simulink model "Copy_of_eCS_Algo_Simulation_2015b"  (R2015b)
settings: Solver=ode1  StartTime=0.0  StopTime=3  FixedStep=1/80000  RelTol=1e-3
PreLoadFcn:
  | if exist('tl_preloadfcn','file'), tl_preloadfcn(gcs,402); end
PostLoadFcn:
  | , if any(exist('dsrtsu_mdlpostloadfcn', 'file') == [2, 3, 6]), try dsrtsu_mdlpostloadfcn('Execute', bdroot); catch fprintf('Error in PostLoadFcn (dsrtsu_mdlpostloadfcn) for model "%s":\n %s\n', bdroot, lasterr); end, end,
  | if exist('tl_postloadfcn','file'), tl_postloadfcn(gcs,402); end
InitFcn:
  | if exist('tlds_init','file'), tlds_init(gcs); end
StartFcn:
  | if exist('tlds_start','file'), tlds_start(gcs); end
StopFcn:
  | if exist('tlds_stop','file'), tlds_stop(gcs); end
model workspace (MAT data in the model file):
  au8PrevExecProfile = [0 0 0 0 0 0]
values from neighbouring files (symbols this model uses):
  AccSensor = 5    [Parameter_eCS_Algo.m]
  AlgoType = 0    [Parameter_eCS_Algo.m]
  Cxy = 1*0.017    (= 0.017)    [Acc_Init_SelV1.m]
  Cxz = 1*0.017    (= 0.017)    [Acc_Init_SelV1.m]
  Cyx = 1*0.017    (= 0.017)    [Acc_Init_SelV1.m]
  Cyz = 1*0.017    (= 0.017)    [Acc_Init_SelV1.m]
  Czx = 1*0.017    (= 0.017)    [Acc_Init_SelV1.m]
  Czy = 1*0.017    (= 0.017)    [Acc_Init_SelV1.m]
  Forced_Oscillation = 0    [Parameter_eCS_Algo.m]    (also in run_Rotation_sim.m = run)
  FreqTemperature = 10    [Acc_Init_SelV1.m]
  MaxSensorOffset = 0.3    [Acc_Init_SelV1.m]
  Mean_x_noise = 4e-3    (= 0.004)    [Acc_Init_SelV1.m]
  Mean_y_noise = 4e-3    (= 0.004)    [Acc_Init_SelV1.m]
  Mean_z_noise = 4e-3    (= 0.004)    [Acc_Init_SelV1.m]
  ODR = 8000    [Acc_Init_SelV1.m]
  offsetcorrection_on_off = 0    [Parameter_eCS_Algo.m]
  phi_pulse_rotation = 0    [Parameter_eCS_Algo.m]    (also in run_Rotation_sim.m = angle)
  pulsetype = 2    [Parameter_eCS_Algo.m]    (also in run_simulation.m = j; run_simulation_ActiveX.m = j)
  Range = 4    [Acc_Init_SelV1.m]
  TempBias = 0    [Acc_Init_SelV1.m]
  TemperatureAmp = 0    [Acc_Init_SelV1.m]
  Var_x_noise = 1.84e-9    (= 1.84e-09)    [Acc_Init_SelV1.m]
  Var_y_noise = 2.025e-09    [Acc_Init_SelV1.m]
  Var_z_noise = 1.374e-09    [Acc_Init_SelV1.m]
  w_x = 2*pi*F_x    (= 376.991118431)    [Acc_Init_SelV1.m]
  w_y = 2*pi*F_y    (= 376.991118431)    [Acc_Init_SelV1.m]
  w_z = 2*pi*F_z    (= 376.991118431)    [Acc_Init_SelV1.m]
  x_max_temp_drift = 0.061    [Acc_Init_SelV1.m]
  x_offset_enable = 0    [Acc_Init_SelV1.m]
  x_run_to_run_drift = 0.0    (= 0)    [Acc_Init_SelV1.m]
  x_temp_co_drift = 0.000    (= 0)    [Acc_Init_SelV1.m]
  Xi_x = 0.7    [Acc_Init_SelV1.m]
  Xi_y = 0.7    [Acc_Init_SelV1.m]
  Xi_z = 0.7    [Acc_Init_SelV1.m]
  y_max_temp_drift = 0.061    [Acc_Init_SelV1.m]
  y_offset_enable = 0    [Acc_Init_SelV1.m]
  y_run_to_run_drift = 0.0    (= 0)    [Acc_Init_SelV1.m]
  y_temp_co_drift = 0.000    (= 0)    [Acc_Init_SelV1.m]
  z_max_temp_drift = 0.13    [Acc_Init_SelV1.m]
  z_offset_enable = 0    [Acc_Init_SelV1.m]
  z_run_to_run_drift = 0.0    (= 0)    [Acc_Init_SelV1.m]
  z_temp_co_drift = 0.000    (= 0)    [Acc_Init_SelV1.m]
undefined symbols (not defined in the file or in its folder): controller_sample_rate, ddv, DiscIntNeverNeededParam, ECE_L_0_x, ECE_L_0_y, ECE_L_0_z, ECE_L_45_time, ECE_L_45_x, ECE_L_45_y, ECE_L_45_z, FMVSS_45_time, FMVSS_45_x, FMVSS_45_y, FMVSS_45_z, gmw_roada_x__m_s__, gmw_roada_y__m_s__, gmw_roadtime_2kHz, KSF_50_a_x, KSF_50_a_y, KSF_50_time, KSG_30_a_x, KSG_30_a_y, KSG_30_time, Meldorf_HindenburgstraAcceleration_x__m_s_2_, Meldorf_HindenburgstraAcceleration_y__m_s_2_, Meldorf_HindenburgstraAcceleration_z__m_s_2_, Meldorf_HindenburgstraTime__s_, pulse_FF27, pulse_MPDB, pulse_ODB40, pulse_ODB64, pulse_USNCAP, pulsetime_FF27, pulsetime_MPDB, pulsetime_ODB40, pulsetime_ODB64, pulsetime_USNCAP, Rauasphalt_60_a_x, Rauasphalt_60_a_y, Rauasphalt_60_time, sigbuilder_block, TimeArray, VW_416_2kHza_x_2kHz, VW_416_2kHza_y_2kHz, VW_416_2kHztime_2kHz
libraries: simulink x40, tllib x10, tl_autosar_lib x7, simulink_extras x5, LIB_TF_G_111 x2, LIB_TF_G_12_StepControl x2, LIB_TF_G_112 x1, dspsigops x1
(part 2 of 9)

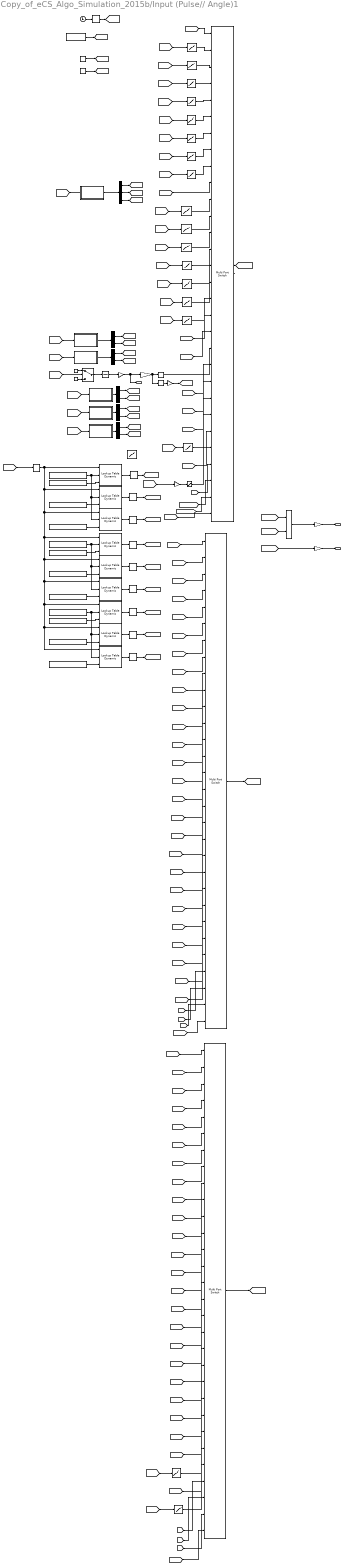
== system Copy_of_eCS_Algo_Simulation_2015b/Input (Pulse// Angle)1 ==
  note: pulse tables must begin and end with 0 !!!!!!!
  -1.0 : Constant  Value=-1
  BMW QV72003-3 no-fire lower : Lookup_n-D  NumberOfTableDimensions=1  BreakpointsForDimension1=[-0.011 0.00 0.020 0.045 0.059]  Table=[0 0 11.0 11.0 0]  ExtrapMethod=Clip  UseLastTableValue=on  InternalRulePriority=Speed  RndMeth=Simplest  InputSameDT=on
  BMW QV72003-3 no-fire upper : Lookup_n-D  NumberOfTableDimensions=1  BreakpointsForDimension1=[0 0.027 0.059 0.085]  Table=[0 16.2 16.2 0]  ExtrapMethod=Clip  UseLastTableValue=on  InternalRulePriority=Speed  RndMeth=Simplest  InputSameDT=on
  Clock : Clock
  Constant : Constant  Value=TimeArray
  Constant1 : Constant  Value=ECE_L_0_x
  Constant10 : Constant  Value=FMVSS_45_z
  Constant11 : Constant  Value=FMVSS_45_y
  Constant2 : Constant  Value=ECE_L_0_z
  Constant3 : Constant  Value=ECE_L_0_y
  Constant4 : Constant  Value=ECE_L_45_time
  Constant5 : Constant  Value=ECE_L_45_x
  Constant6 : Constant  Value=ECE_L_45_z
  Constant7 : Constant  Value=ECE_L_45_y
  Constant8 : Constant  Value=FMVSS_45_time
  Constant9 : Constant  Value=FMVSS_45_x
  Demux1 : Demux  Outputs=3
  Demux{2..6} (5 alike) : Demux  Outputs=2
  Discrete-Time Integrator4 : DiscreteIntegrator  gainval=1  InitialConditionSetting=State (most efficient)  SampleTime=-1  UpperSaturationLimit=0.3 * 9.81  LowerSaturationLimit=-0.3 * 9.81  ICPrevOutput=DiscIntNeverNeededParam  ICPrevScaledInput=DiscIntNeverNeededParam
  Gain : Gain  Gain=-1
  Lookup Table Dynamic{,1..8} (9 alike) : simulink/Lookup Tables/Lookup Table Dynamic  LookUpMeth=Interpolation-Use End Values  OutDataTypeStr=fixdt('double')  OutputDataTypeScalingMode=Specify via dialog  OutDataType=fixdt('double')  OutScaling=[]  DoSatur=off
  Multiport Switch1 : MultiPortSwitch  Inputs=28  DataPortForDefault=Additional data port
  Multiport Switch2 : MultiPortSwitch  Inputs=28  DataPortForDefault=Additional data port
  Multiport Switch3 : MultiPortSwitch  Inputs=28  DataPortForDefault=Additional data port
  Mux1 : Mux  Inputs=2
  Puls_BMW_KSF_50 : Subsystem
  Puls_BMW_KSG_30 : Subsystem
  "Puls_BMW_Rauasphalt_60 " : Subsystem
  Puls_GWM_road_C.Morgan : Subsystem
  Puls_Kopfsteinpflaster Meldorf Hindenburgstrasse : Subsystem
  Puls_VW416_Atlas_C.Morgan : Subsystem
  Pulse table FF27 (g) : Lookup  InputValues=pulsetime_FF27  Table=pulse_FF27  LookUpMeth=Interpolation-Use End Values
  Pulse table MPDB (g) : Lookup  InputValues=pulsetime_MPDB  Table=pulse_MPDB  LookUpMeth=Interpolation-Use End Values
  Pulse table ODB40 (g) : Lookup  InputValues=pulsetime_ODB40  Table=pulse_ODB40  LookUpMeth=Interpolation-Use End Values
  Pulse table ODB64 (g) : Lookup  InputValues=pulsetime_ODB64  Table=pulse_ODB64  LookUpMeth=Interpolation-Use End Values
  Pulse table USNCAP (g) : Lookup  InputValues=pulsetime_USNCAP  Table=pulse_USNCAP  LookUpMeth=Interpolation-Use End Values
  Rate Transition{,1,3..10} (10 alike) : RateTransition
  Rate Transition2 : RateTransition  OutPortSampleTime=1/2000
  Saturation : Saturate  UpperLimit=5  LowerLimit=0
  Sin1 : Trigonometry  Operator=cos
  Sin2 : Trigonometry
  Switch : Switch  Criteria=u2 > Threshold  Threshold=36
  crash angle in rad : Gain  Gain=2*pi/360
  g in m/s² : Gain  Gain=9.807
  g in m/s²1 : Gain  Gain=9.807
  "g-lock \" must lock\" - 6g/s - 0.45g" : Lookup_n-D  NumberOfTableDimensions=1  BreakpointsForDimension1=[0 0.075 0.3 0.4]  Table=[0 0.45 0.45 0]  ExtrapMethod=Clip  UseLastTableValue=on  InternalRulePriority=Speed  RndMeth=Simplest  InputSameDT=on
  "g-lock \" no lock\" - 6g/s - 0.3g" : Lookup_n-D  NumberOfTableDimensions=1  BreakpointsForDimension1=[0 0.050 0.5 0.6]  Table=[0 0.3 0.3 0]  ExtrapMethod=Clip  UseLastTableValue=on  InternalRulePriority=Speed  RndMeth=Simplest  InputSameDT=on
  g-lock Crash - 2000g/s - 30g : Lookup_n-D  NumberOfTableDimensions=1  BreakpointsForDimension1=[0 0.015 0.055 0.08]  Table=[0 30 30 0]  ExtrapMethod=Clip  UseLastTableValue=on  InternalRulePriority=Speed  RndMeth=Simplest  InputSameDT=on
  g-lock ECE - 150g/s - 0.45g : Lookup_n-D  NumberOfTableDimensions=1  BreakpointsForDimension1=[0 0.003 0.3 0.4]  Table=[0 0.45 0.45 0]  ExtrapMethod=Clip  UseLastTableValue=on  InternalRulePriority=Speed  RndMeth=Simplest  InputSameDT=on
  g-lock ECE - 25g/s - 0.45g : Lookup_n-D  NumberOfTableDimensions=1  BreakpointsForDimension1=[0 0.018 0.3 0.4]  Table=[0 0.45 0.45 0]  ExtrapMethod=Clip  UseLastTableValue=on  InternalRulePriority=Speed  RndMeth=Simplest  InputSameDT=on
  g-lock ECE - 25g/s - 0.45g custom : Lookup_n-D  NumberOfTableDimensions=1  BreakpointsForDimension1=[0 0.1 0.10001 1]  Table=[0 0 1 1]  ExtrapMethod=Clip  UseLastTableValue=on  InternalRulePriority=Speed  RndMeth=Simplest  InputSameDT=on
  g-lock ECE - 25g/s - 0.45g custom1 : Lookup_n-D  NumberOfTableDimensions=1  BreakpointsForDimension1=[0,0.018,0.3,0.4,0.6,0.618,1,1.1,3,3.018,3.05,3.1,3.118,3.5,3.6,4,4.018,4.2,4.3,8,8.018,8.1,8.15,9,9.018,9.3,9.4,10]  Table=[0,0.45,0.45,0,0,0.45,0.45,0,0,0.45,0.45,0,0.45,0.45,0,0,0.45,0.45,0,0,0.45,0.45,0,0,0.45,0.45,0,0]  ExtrapMethod=Clip  UseLastTableValue=on  InternalRulePriority=Speed  RndMeth=Simplest  InputSameDT=on
  g-lock FMVSS  - 16g/s - 0,7g : Lookup_n-D  NumberOfTableDimensions=1  BreakpointsForDimension1=[0 0.04375 0.3 0.4]  Table=[0 0.7 0.7 0]  ExtrapMethod=Clip  UseLastTableValue=on  InternalRulePriority=Speed  RndMeth=Simplest  InputSameDT=on
  g-lock FMVSS - 70g/s - 0.7g : Lookup_n-D  NumberOfTableDimensions=1  BreakpointsForDimension1=[0 0.01 0.3 0.4]  Table=[0 0.7 0.7 0]  ExtrapMethod=Clip  UseLastTableValue=on  InternalRulePriority=Speed  RndMeth=Simplest  InputSameDT=on
  g-lock Vollbremsung - 4g/s - 1g : Lookup_n-D  NumberOfTableDimensions=1  BreakpointsForDimension1=[0 0.25 0.9745 1.2]  Table=[0 1 1 0]  ExtrapMethod=Clip  UseLastTableValue=on  InternalRulePriority=Speed  RndMeth=Simplest  InputSameDT=on
  g_rate : Gain  Gain=5
  generic rollover : Lookup_n-D  NumberOfTableDimensions=1  BreakpointsForDimension1=[0 15 16 20 25 30 30.001 32 35 60]  Table=[-1 -1 1 1 0.5 0.5 0.49 0.49 -1 -1]  ExtrapMethod=Clip  UseLastTableValue=on  InternalRulePriority=Speed  RndMeth=Simplest  InputSameDT=on
  pulsetype : Constant  Value=pulsetype
  rollover ? : Lookup_n-D  NumberOfTableDimensions=1  BreakpointsForDimension1=[0 0.01 0.39 0.4]  Table=[0 1 1 0]  ExtrapMethod=Clip  UseLastTableValue=on  InternalRulePriority=Speed  RndMeth=Simplest  InputSameDT=on
  tilt speed : Gain  Gain=10
  time_const : Constant  Value=-1
  time_const1 : Constant
  zero : Constant  Value=0.0
  "Pulse_profile " : Outport
  Pulse z-axis : Outport  Port=2
  angle in ° : Outport  Port=3
  wires:
  crash angle in rad/1 -> Sin1/1, Sin2/1
  tilt speed/1 -> angle in °/1, crash angle in rad/1
  time_const1/1 -> Switch/3
  time_const/1 -> Switch/1
  Switch/1 -> Discrete-Time Integrator4/1
  Discrete-Time Integrator4/1 -> tilt speed/1
  g_rate/1 -> Saturation/1
  Mux1/1 -> g in m/s²/1
  g in m/s²/1 -> "Pulse_profile "/1
  Clock/1 -> Rate Transition/1
  [time] -> g-lock ECE - 150g/s - 0.45g/1
  [time] -> g-lock ECE - 25g/s - 0.45g/1
  [time] -> g-lock FMVSS  - 16g/s - 0,7g/1
  Rate Transition/1 -> [time]
  [time] -> g-lock FMVSS - 70g/s - 0.7g/1
  [time] -> "g-lock \" no lock\" - 6g/s - 0.3g"/1
  [time] -> "g-lock \" must lock\" - 6g/s - 0.45g"/1
  [time] -> g-lock Vollbremsung - 4g/s - 1g/1
  [time] -> g-lock Crash - 2000g/s - 30g/1
  [time] -> Pulse table USNCAP (g)/1
  [time] -> Switch/2
  [time] -> g_rate/1
  [time] -> Puls_Kopfsteinpflaster Meldorf Hindenburgstrasse/1(time in)
  pulsetype/1 -> [pulsetype]
  [pulsetype] -> Multiport Switch3/1
  [pulsetype] -> Multiport Switch2/1
  Puls_Kopfsteinpflaster Meldorf Hindenburgstrasse/1(pulse out [x,y] (g)) -> Demux1/1
  Demux1/1 -> [x_09]
  Demux1/2 -> [y_09]
  zero/1 -> [zero]
  [zero] -> Multiport Switch2/2
  [zero] -> Multiport Switch2/3
  [zero] -> Multiport Switch2/4
  [zero] -> Multiport Switch2/5
  [zero] -> Multiport Switch2/6
  [zero] -> Multiport Switch2/7
  [zero] -> Multiport Switch2/8
  [zero] -> Multiport Switch2/9
  [zero] -> Multiport Switch2/12
  [zero] -> Multiport Switch2/13
  [zero] -> Multiport Switch2/14
  [y_09] -> Multiport Switch2/10
  [zero] -> Multiport Switch2/11
  [y_17] -> Multiport Switch2/18
  [zero] -> Multiport Switch2/17
  [zero] -> Multiport Switch2/16
  [zero] -> Multiport Switch2/15
  [y_18] -> Multiport Switch2/19
  [zero] -> Multiport Switch2/20
  [time] -> Pulse table FF27 (g)/1
  [time] -> Pulse table ODB40 (g)/1
  [time] -> Pulse table ODB64 (g)/1
  [time] -> Pulse table MPDB (g)/1
  [time] -> BMW QV72003-3 no-fire upper/1
  [time] -> BMW QV72003-3 no-fire lower/1
  Demux2/2 -> [y_17]
  Demux2/1 -> [x_17]
  Puls_GWM_road_C.Morgan/1(pulse out [x,y] (g)) -> Demux2/1
  [time] -> Puls_GWM_road_C.Morgan/1(time in)
  Puls_VW416_Atlas_C.Morgan/1(pulse out [x,y] (g)) -> Demux3/1
  Demux3/1 -> [x_18]
  Demux3/2 -> [y_18]
  [time] -> Puls_VW416_Atlas_C.Morgan/1(time in)
  Saturation/1 -> Multiport Switch3/26
  g-lock ECE - 25g/s - 0.45g/1 -> Multiport Switch3/3
  g-lock FMVSS  - 16g/s - 0,7g/1 -> Multiport Switch3/4
  g-lock ECE - 150g/s - 0.45g/1 -> Multiport Switch3/2
  g-lock FMVSS - 70g/s - 0.7g/1 -> Multiport Switch3/5
  "g-lock \" no lock\" - 6g/s - 0.3g"/1 -> Multiport Switch3/6
  "g-lock \" must lock\" - 6g/s - 0.45g"/1 -> Multiport Switch3/7
  g-lock Vollbremsung - 4g/s - 1g/1 -> Multiport Switch3/8
  g-lock Crash - 2000g/s - 30g/1 -> Multiport Switch3/9
  [x_09] -> Multiport Switch3/10
  Pulse table USNCAP (g)/1 -> Multiport Switch3/11
  Pulse table FF27 (g)/1 -> Multiport Switch3/12
  Pulse table ODB40 (g)/1 -> Multiport Switch3/13
  Pulse table ODB64 (g)/1 -> Multiport Switch3/14
  Pulse table MPDB (g)/1 -> Multiport Switch3/15
  BMW QV72003-3 no-fire upper/1 -> Multiport Switch3/16
  BMW QV72003-3 no-fire lower/1 -> Multiport Switch3/17
  [x_17] -> Multiport Switch3/18
  [x_18] -> Multiport Switch3/19
  Sin2/1 -> Multiport Switch3/20
  [zero] -> Multiport Switch2/26
  [zero] -> Multiport Switch2/25
  [y_09] -> Multiport Switch2/24
  [y_20] -> Multiport Switch2/21
  [y_21] -> Multiport Switch2/22
  [y_22] -> Multiport Switch2/23
  [x_20] -> Multiport Switch3/21
  [x_22] -> Multiport Switch3/23
  [x_21] -> Multiport Switch3/22
  Puls_BMW_KSF_50/1(pulse out [x,y] (g)) -> Demux4/1
  [time] -> Puls_BMW_KSF_50/1(time in)
  Demux4/1 -> [x_20]
  Demux4/2 -> [y_20]
  [time] -> Puls_BMW_KSG_30/1(time in)
  Puls_BMW_KSG_30/1(pulse out [x,y] (g)) -> Demux5/1
  Demux5/1 -> [x_21]
  Demux5/2 -> [y_21]
  "Puls_BMW_Rauasphalt_60 "/1(pulse out [x,y] (g)) -> Demux6/1
  [time] -> "Puls_BMW_Rauasphalt_60 "/1(time in)
  Demux6/1 -> [x_22]
  Demux6/2 -> [y_22]
  [minus_one] -> Multiport Switch1/23
  [minus_one] -> Multiport Switch1/22
  [minus_one] -> Multiport Switch1/21
  generic rollover/1 -> Multiport Switch1/24
  [minus_one] -> Multiport Switch1/25
  rollover ?/1 -> Multiport Switch1/26
  [z_19] -> Multiport Switch1/20
  [minus_one] -> Multiport Switch1/19
  [minus_one] -> Multiport Switch1/15
  [minus_one] -> Multiport Switch1/16
  [minus_one] -> Multiport Switch1/17
  [minus_one] -> Multiport Switch1/18
  [minus_one] -> Multiport Switch1/11
  [z_09] -> Multiport Switch1/10
  [minus_one] -> Multiport Switch1/14
  [minus_one] -> Multiport Switch1/13
  [minus_one] -> Multiport Switch1/12
  [minus_one] -> Multiport Switch1/9
  [minus_one] -> Multiport Switch1/8
  [minus_one] -> Multiport Switch1/7
  [minus_one] -> Multiport Switch1/6
  [minus_one] -> Multiport Switch1/5
  [minus_one] -> Multiport Switch1/4
  [minus_one] -> Multiport Switch1/3
  [minus_one] -> Multiport Switch1/2
  [pulsetype] -> Multiport Switch1/1
  Multiport Switch1/1 -> [z_acceleration]
  Multiport Switch2/1 -> [y_acceleration]
  [y_acceleration] -> Mux1/2  "ay(g)"
  [x_acceleration] -> Mux1/1  "ax(g)"
  Multiport Switch3/1 -> [x_acceleration]
  [z_acceleration] -> g in m/s²1/1  "az(g)"
  [time] -> rollover ?/1
  -1.0/1 -> [minus_one]
  g in m/s²1/1 -> Pulse z-axis/1
  Demux1/3 -> [z_09]
  Sin1/1 -> Gain/1
  Gain/1 -> [z_19]
  [time] -> generic rollover/1
  [time] -> g-lock ECE - 25g/s - 0.45g custom/1
  [x_09] -> Multiport Switch3/25
  g-lock ECE - 25g/s - 0.45g custom/1 -> Multiport Switch3/24
  [time] -> Rate Transition2/1
  Constant1/1 -> Lookup Table Dynamic/3
  Constant3/1 -> Lookup Table Dynamic1/3
  Constant/1 -> Lookup Table Dynamic2/2, Lookup Table Dynamic1/2, Lookup Table Dynamic/2
  Constant2/1 -> Lookup Table Dynamic2/3
  Constant5/1 -> Lookup Table Dynamic3/3
  Constant7/1 -> Lookup Table Dynamic4/3
  Constant4/1 -> Lookup Table Dynamic5/2, Lookup Table Dynamic4/2, Lookup Table Dynamic3/2
  Constant6/1 -> Lookup Table Dynamic5/3
  Lookup Table Dynamic/1 -> Rate Transition1/1
  Lookup Table Dynamic1/1 -> Rate Transition3/1
  Lookup Table Dynamic2/1 -> Rate Transition4/1
  Lookup Table Dynamic3/1 -> Rate Transition5/1
  Lookup Table Dynamic4/1 -> Rate Transition6/1
  Lookup Table Dynamic5/1 -> Rate Transition7/1
  [ECE_L_0_x] -> Multiport Switch3/27
  [ECE_L_45_x] -> Multiport Switch3/28
  [ECE_L_0_y] -> Multiport Switch2/27
  [ECE_L_45_y] -> Multiport Switch2/28
  [ECE_L_0_z] -> Multiport Switch1/27
  [ECE_L_45_z] -> Multiport Switch1/28
  Rate Transition1/1 -> [ECE_L_0_x]
  Rate Transition3/1 -> [ECE_L_0_y]
  Rate Transition4/1 -> [ECE_L_0_z]
  Rate Transition5/1 -> [ECE_L_45_x]
  Rate Transition6/1 -> [ECE_L_45_y]
  Rate Transition7/1 -> [ECE_L_45_z]
  Rate Transition2/1 -> Lookup Table Dynamic6/1, Lookup Table Dynamic7/1, Lookup Table Dynamic8/1, Lookup Table Dynamic5/1, Lookup Table Dynamic4/1, Lookup Table Dynamic3/1, Lookup Table Dynamic2/1, Lookup Table Dynamic1/1, Lookup Table Dynamic/1
  Constant9/1 -> Lookup Table Dynamic6/3
  Constant11/1 -> Lookup Table Dynamic7/3
  Constant8/1 -> Lookup Table Dynamic6/2, Lookup Table Dynamic7/2, Lookup Table Dynamic8/2
  Constant10/1 -> Lookup Table Dynamic8/3
  Lookup Table Dynamic6/1 -> Rate Transition8/1
  Lookup Table Dynamic7/1 -> Rate Transition9/1
  Lookup Table Dynamic8/1 -> Rate Transition10/1
  Rate Transition8/1 -> [FMVSS_45_x]
  Rate Transition9/1 -> [FMVSS_45_y]
  Rate Transition10/1 -> [FMVSS_45_z]
  [zero] -> Multiport Switch2/30
  [FMVSS_45_y] -> Multiport Switch2/29
  [minus_one] -> Multiport Switch1/30
  [FMVSS_45_z] -> Multiport Switch1/29
  [zero] -> Multiport Switch3/30
  [FMVSS_45_x] -> Multiport Switch3/29

== system Copy_of_eCS_Algo_Simulation_2015b/Noisy ==
  Demux : Demux  Tag=STV Demux  Outputs=1
  FromWs : FromWorkspace  Tag=STV FromWs  VariableName=tuvar  SampleTime=0
      SigBuilderData=|
      | common.afterFinalStr = 'Extrapolate'
      | common.sampleTime = 0
      | dataSet.timeRange = [0 0.01]
      | dataSet.name = 'Group 1'
      | sbobj.Groups.Name = 'Group 1'
      | sbobj.Groups.Signals.Name = 'Signal 1'
      | sbobj.Groups.Signals.XData = [0 0.0005 0.001 0.001 0.0015 0.0015 0.002 0.002 0.0025 0.0025 0.003 0.003 0.0035 0.0035 0.004 0.004 0.0045 0.0045 0.005 0.005 0.0055 0.0055 0.006 0.006 0.0065 0.007 0.007 0.0075 0.0075 0.008 0.008 0.0085 0.009 0.0095 0.0095 0.01]
      | sbobj.Groups.Signals.YData = [0 0 1.26 0.79 0.8 0.02 0.02 1.11 1.11 0.8 0.8 0 0 -0.02 1 0.02 0.005 0 0.63 0.65 0.9 0.22 1.09 0.04 0.4 1.58 1.18 1.12 0.32 0.8 0 -0.02 1.12 -0.02 0 0]
      | sbobj.Groups.TimeRange = [0 0.01]
  Signal 1 : Outport  Tag=STV Outport
  wires:
  FromWs/1 -> Demux/1
  Demux/1 -> Signal 1/1

== system Copy_of_eCS_Algo_Simulation_2015b/SAD ==
  prrFsmProfile : Inport
  Subsystem : Subsystem  Tag=struct('sfcnName','SAD_sf','subFunction','','srcSubsystem','')  mask(TL_Enable){}
      settings: OpenFcn=warndlg(get_param(gcb,'MaskHelp'),'Serious Warning');
      mask Help: This subsystem keeps the TargetLink subsystem (subsystem with TargetLink blocks for production code generation), and is needed for the TargetLink simulation frame to work properly. DO NOT DELETE OR MODIFY IT!
  psrExecutedProfiles : Outport
  wires:
  prrFsmProfile/1 -> Subsystem/1(prrFsmProfile)
  Subsystem/1(psrExecutedProfiles) -> psrExecutedProfiles/1

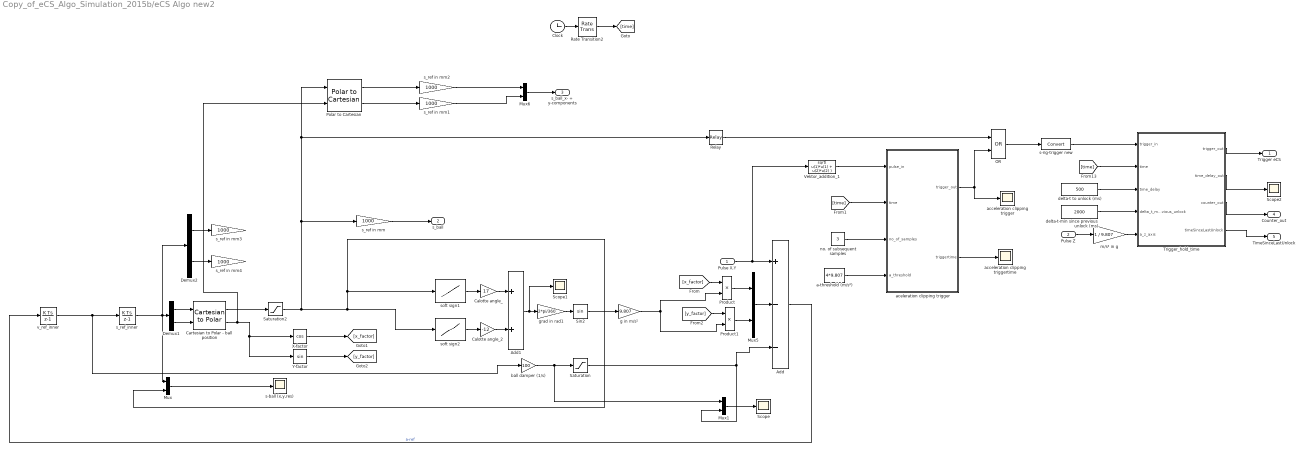
== system Copy_of_eCS_Algo_Simulation_2015b/eCS Algo new2 ==
  Pulse X,Y : Inport
  Pulse Z : Inport  Port=2
  Add : Sum  Inputs=+--
  Add1 : Sum
  Calotte angle_ : Gain  Gain=17
  Calotte angle_2 : Gain  Gain=-12
  Cartesian to Polar - ball position : simulink_extras/Transformations/Cartesian to Polar
  Clock : Clock
  Demux1 : Demux  Outputs=2
  Demux2 : Demux  Outputs=2
  Mux{,1,5..6} (4 alike) : Mux  Inputs=2
  OR : Logic  Operator=OR  AllPortsSameDT=off  OutDataTypeStr=boolean
  Polar to Cartesian : simulink_extras/Transformations/Polar to Cartesian
  Product : Product
  Product1 : Product
  Rate Transition2 : RateTransition
  Relay : Relay  OnSwitchValue=0.0004  OffSwitchValue=0.0001
  Saturation : Saturate  UpperLimit=50  LowerLimit=-50
  Saturation2 : Saturate  UpperLimit=0.001  LowerLimit=0
  Scope : Scope
  Scope1 : Scope
  Scope2 : Scope
  Sin2 : Trigonometry
  Trigger_hold_time : MATLAB Function  TreatAsAtomicUnit=on
  Vektor_addition_1 : Fcn  Expr=sqrt( u(1)*u(1) + u(2)*u(2) )
  X-factor : Trigonometry  Operator=cos
  Y-factor : Trigonometry
  a-threshold (m/s²) : Constant  Value=4*9.807
  acceleration clipping trigger : Scope
  acceleration clipping triggertime : Scope
  aceleration clipping trigger : MATLAB Function  TreatAsAtomicUnit=on
  ball damper (1/s) : Gain  Gain=100
  delta-t to unlock (ms) : Constant  Value=500  OutMin=[0]
  delta-t-min since previous unlock (ms) : Constant  Value=2000  OutMin=[0]
  g in m/s² : Gain  Gain=9.807
  grad in rad1 : Gain  Gain=2*pi/360
  m/s² in g : Gain  Gain=1 / 9.807
  no. of subsequent samples : Constant  Value=3
  s-ball (x,y,res) : Scope
  s-rig-trigger new : DataTypeConversion
  s_ref in mm{,1..4} (5 alike) : Gain  Gain=1000
  s_ref_inner : DiscreteIntegrator  InitialConditionSetting=State (most efficient)  SampleTime=-1  LimitOutput=on  UpperSaturationLimit=0.001  LowerSaturationLimit=-0.001  ICPrevOutput=DiscIntNeverNeededParam  ICPrevScaledInput=DiscIntNeverNeededParam
  soft sign1 : Lookup_n-D  NumberOfTableDimensions=1  BreakpointsForDimension1=[0 0.00002 0.002]  Table=[0 1 1]  ExtrapMethod=Clip  UseLastTableValue=on  InternalRulePriority=Speed  RndMeth=Simplest  InputSameDT=on
  soft sign2 : Lookup_n-D  NumberOfTableDimensions=1  BreakpointsForDimension1="[0 0.0004 0.0005  0.001]"  Table="[0  0 1 1]"  ExtrapMethod=Clip  UseLastTableValue=on  InternalRulePriority=Speed  RndMeth=Simplest  InputSameDT=on
  v_ref_inner : DiscreteIntegrator  InitialConditionSetting=State (most efficient)  SampleTime=-1  ICPrevOutput=DiscIntNeverNeededParam  ICPrevScaledInput=DiscIntNeverNeededParam
  Trigger eCS : Outport
  s_ball : Outport  Port=2
  s_ball_x- + y-components : Outport  Port=3
  Counter_out : Outport  Port=4
  TimeSinceLastUnlock : Outport  Port=5
  wires:
  v_ref_inner/1 -> s_ref_inner/1, ball damper (1/s)/1
  grad in rad1/1 -> Sin2/1
  soft sign1/1 -> Calotte angle_/1
  Calotte angle_/1 -> Add1/1
  soft sign2/1 -> Calotte angle_2/1
  Calotte angle_2/1 -> Add1/2
  Add1/1 -> Scope1/1, grad in rad1/1
  Sin2/1 -> g in m/s²/1
  Cartesian to Polar - ball position/1 -> Saturation2/1
  Pulse X,Y/1 -> Vektor_addition_1/1, Add/1
  ball damper (1/s)/1 -> Mux1/1, Saturation/1
  s_ref in mm/1 -> s_ball/1
  Add/1 -> v_ref_inner/1  "a-ref"
  Mux/1 -> s-ball (x,y,res)/1
  Saturation/1 -> Add/3, Mux1/2
  Mux1/1 -> Scope/1
  Clock/1 -> Rate Transition2/1
  aceleration clipping trigger/2(triggertime) -> acceleration clipping triggertime/1
  no. of subsequent samples/1 -> aceleration clipping trigger/3(no_of_samples)
  a-threshold (m/s²)/1 -> aceleration clipping trigger/4(a_threshold)
  aceleration clipping trigger/1(trigger_out) -> acceleration clipping trigger/1, OR/2
  Relay/1 -> OR/1
  Vektor_addition_1/1 -> aceleration clipping trigger/1(pulse_in)
  [time] -> Trigger_hold_time/2(time)
  Rate Transition2/1 -> [time]
  [time] -> aceleration clipping trigger/2(time)
  delta-t to unlock (ms)/1 -> Trigger_hold_time/3(time_delay)
  OR/1 -> s-rig-trigger new/1
  s-rig-trigger new/1 -> Trigger_hold_time/1(trigger_in)
  delta-t-min since previous unlock (ms)/1 -> Trigger_hold_time/4(delta_t_min_since_previous_unlock)
  Trigger_hold_time/1(trigger_out) -> Trigger eCS/1
  Trigger_hold_time/2(time_delay_out) -> Scope2/1
  Demux1/2 -> Cartesian to Polar - ball position/2
  Demux1/1 -> Cartesian to Polar - ball position/1
  s_ref_inner/1 -> Demux2/1, Mux/1, Demux1/1
  Cartesian to Polar - ball position/2 -> Polar to Cartesian/2, Y-factor/1, X-factor/1
  Mux5/1 -> Add/2
  Product/1 -> Mux5/1
  Product1/1 -> Mux5/2
  g in m/s²/1 -> Product1/2, Product/2
  [x_factor] -> Product/1
  [y_factor] -> Product1/1
  X-factor/1 -> [x_factor]
  Y-factor/1 -> [y_factor]
  Saturation2/1 -> soft sign2/1, soft sign1/1, Mux/2, Polar to Cartesian/1, Relay/1, s_ref in mm/1
  Demux2/1 -> s_ref in mm3/1
  Demux2/2 -> s_ref in mm4/1
  Polar to Cartesian/2 -> s_ref in mm1/1
  Polar to Cartesian/1 -> s_ref in mm2/1
  Mux6/1 -> s_ball_x- + y-components/1
  s_ref in mm1/1 -> Mux6/2
  s_ref in mm2/1 -> Mux6/1
  Pulse Z/1 -> m/s² in g/1
  m/s² in g/1 -> Trigger_hold_time/5(a_z_axis)
  Trigger_hold_time/3(counter_out) -> Counter_out/1
  Trigger_hold_time/4(timeSinceLastUnlock) -> TimeSinceLastUnlock/1

== system Copy_of_eCS_Algo_Simulation_2015b/eCS_Targetlink ==
  note: SIL Fixed-point
  note: MIL Floating point
  Ax (m.s-2) : Inport
  Ay (m.s-2) : Inport  Port=2
  Az (m.s-2) : Inport  Port=3
  Subsystem : Subsystem  Tag=struct('sfcnName','eCS_Targetlink_sf','subFunction','','srcSubsystem','')  mask(TL_Enable){}
      settings: OpenFcn=warndlg(get_param(gcb,'MaskHelp'),'Serious Warning');
      mask Help: This subsystem keeps the TargetLink subsystem (subsystem with TargetLink blocks for production code generation), and is needed for the TargetLink simulation frame to work properly. DO NOT DELETE OR MODIFY IT!
  sBall : Outport
  b8eCSTrigg : Outport  Port=2
  wires:
  Ax (m.s-2)/1 -> Subsystem/1(Ax (m.s-2))
  Ay (m.s-2)/1 -> Subsystem/2(Ay (m.s-2))
  Az (m.s-2)/1 -> Subsystem/3(Az (m.s-2))
  Subsystem/1(sBall) -> sBall/1
  Subsystem/2(b8eCSTrigg) -> b8eCSTrigg/1

== system Copy_of_eCS_Algo_Simulation_2015b/oscilliation generator ==
  bOscillationReq : Inport
  Constant1 : Constant  Value=0
  Constant3 : Constant  Value=0
  Constant5 : Constant  Value=0
  Discrete FIR Filter : DiscreteFir
  Scope : Scope
  Sine Wave : Sin  Amplitude=0.2  Frequency=6280  Phase=3.14/2  SampleTime=0
  Sine Wave2 : Sin  Amplitude=0.2  Frequency=1256  SampleTime=0
  Switch1 : Switch  Criteria=u2 ~= 0
  Switch2 : Switch  Criteria=u2 ~= 0
  Switch3 : Switch  Criteria=u2 ~= 0
  Oscillation_ax : Outport
  Oscillation_ay : Outport  Port=2
  Oscillation_az : Outport  Port=3
  wires:
  Switch1/1 -> Oscillation_ax/1
  Sine Wave/1 -> Scope/1, Switch2/1, Switch1/1
  Constant3/1 -> Switch1/3
  Constant5/1 -> Switch2/3
  Switch2/1 -> Oscillation_ay/1
  Sine Wave2/1 -> Switch3/1
  Constant1/1 -> Switch3/3
  bOscillationReq/1 -> Switch3/2, Switch2/2, Switch1/2
  Switch3/1 -> Oscillation_az/1

== system Copy_of_eCS_Algo_Simulation_2015b/pulse rotation around z-axis ==
  pulse in m/s² : Inport
  rotation angle : Inport  Port=2
  Enable : EnablePort
  Add5 : Sum
  Cartesian to Polar : simulink_extras/Transformations/Cartesian to Polar
  Degrees to Radians : simulink_extras/Transformations/Degrees to Radians
  Demux1 : Demux  Outputs=2
  Mux10 : Mux  Inputs=2
  Polar to Cartesian : simulink_extras/Transformations/Polar to Cartesian
  Scope : Scope  NumInputPorts=2
  pulse rotated in m/s² : Outport
  wires:
  rotation angle/1 -> Degrees to Radians/1
  Degrees to Radians/1 -> Add5/2
  Demux1/2 -> Cartesian to Polar/2
  Add5/1 -> Polar to Cartesian/2
  Cartesian to Polar/1 -> Polar to Cartesian/1
  Demux1/1 -> Cartesian to Polar/1
  Cartesian to Polar/2 -> Add5/1
  Polar to Cartesian/1 -> Mux10/1
  Polar to Cartesian/2 -> Mux10/2
  pulse in m/s²/1 -> Demux1/1
  Mux10/1 -> pulse rotated in m/s²/1  "pulse rotated in m/s²"

== system Copy_of_eCS_Algo_Simulation_2015b/µC Signalverarbeitung und Algorithmus2 ==
  Acceleration x-Axis (g) : Inport
  Acceleration y-Axis (g) : Inport  Port=2
  Acceleration z-Axis (g) : Inport  Port=3
  Bessel Filter x 4th order 50Hz : DiscreteFilter  Numerator=[5.797239396826742e-08 2.318895758730697e-07 3.478343638096045e-07 2.318895758730697e-07 5.797239396826742e-08]  Denominator=[1 -3.902348194587603 5.711314979977801 -3.715489008702718 0.906523150870823]
  Bessel Filter y : DiscreteFilter  Numerator=[5.797239396826742e-08 2.318895758730697e-07 3.478343638096045e-07 2.318895758730697e-07 5.797239396826742e-08]  Denominator=[1 -3.902348194587603 5.711314979977801 -3.715489008702718 0.906523150870823]
  Bessel Filter z : DiscreteFilter  Numerator=[5.797239396826742e-08 2.318895758730697e-07 3.478343638096045e-07 2.318895758730697e-07 5.797239396826742e-08]  Denominator=[1 -3.902348194587603 5.711314979977801 -3.715489008702718 0.906523150870823]
  Calculate Onset >=Threshold : Subsystem
  Logical Operator : Logic  Operator=OR  Inputs=3  AllPortsSameDT=off  OutDataTypeStr=boolean
  Logical Operator1 : Logic  AllPortsSameDT=off  OutDataTypeStr=boolean
  Mux : Mux  Inputs=2
  Oversampling µC z-Axis : ZeroOrderHold  SampleTime=1/10000
  RT : RateTransition  OutPortSampleTime=0.001
  RT1 : RateTransition  OutPortSampleTime=0.0001
  Resulting xy >= Threshold : Subsystem
  Scope : Scope
  Scope1 : Scope  NumInputPorts=4
  Scope2 : Scope
  Terminator : Terminator
  Tilt Sensitivity >= Threshold : Subsystem
  Unit Delay : UnitDelay  SampleTime=1/1000
  no lock / lock [bool] : Outport
  wires:
  Acceleration z-Axis (g)/1 -> Oversampling µC z-Axis/1
  Resulting xy >= Threshold/1(no lock / lock [bool]) -> Logical Operator/1
  Logical Operator1/1 -> Scope2/1, no lock / lock [bool]/1
  Tilt Sensitivity >= Threshold/1(no lock / lock [bool]) -> Logical Operator/2
  Bessel Filter y/1 -> Scope1/4, Resulting xy >= Threshold/2(Acceleration y-Axis corrected [g]), Tilt Sensitivity >= Threshold/2(Acceleration y [g])
  Bessel Filter x 4th order 50Hz/1 -> Scope1/2, Resulting xy >= Threshold/1(Acceleration x-Axis corrected [g]), Tilt Sensitivity >= Threshold/1(Acceleration x [g]), Mux/2
  Unit Delay/1 -> RT1/1
  Oversampling µC z-Axis/1 -> Bessel Filter z/1, Calculate Onset >=Threshold/3(Acceleration z-Axis[g])
  Calculate Onset >=Threshold/1(no lock / lock [bool]) -> Logical Operator/3
  Acceleration y-Axis (g)/1 -> Scope1/3, Bessel Filter y/1, Calculate Onset >=Threshold/2(Acceleration y-Axis[g])
  Acceleration x-Axis (g)/1 -> Scope1/1, Mux/1, Bessel Filter x 4th order 50Hz/1, Calculate Onset >=Threshold/1(Acceleration x-Axis[g])
  Bessel Filter z/1 -> Terminator/1
  Mux/1 -> Scope/1
  Logical Operator/1 -> RT/1, Logical Operator1/1
  RT/1 -> Unit Delay/1
  RT1/1 -> Logical Operator1/2

== system Copy_of_eCS_Algo_Simulation_2015b/FSM/Subsystem ==
  prrEcsAlgoFlag : Inport
  prrVehicleInputs : Inport  Port=2
  prrExecutedProfiles : Inport  Port=3
  FSM : Subsystem  Tag=MIL Subsystem  Description=b  mask(MIL Subsystem){}
      settings: CopyFcn=if exist('tl_copyfcn','file'), tl_copyfcn(gcbh); end  NameChangeFcn=if exist('tl_namechangefcn','file'), tl_namechangefcn(gcbh); end  DestroyFcn=if exist('update_tl_main_dlg','file'), update_tl_main_dlg('TL_subs_display'); end
  psrSolenoidState : Outport
  psrFsmProfile : Outport  Port=2
  wires:
  prrEcsAlgoFlag/1 -> FSM/1(prrEcsAlgoFlag)
  prrVehicleInputs/1 -> FSM/2(prrVehicleInputs)
  prrExecutedProfiles/1 -> FSM/3(prrExecutedProfiles)
  FSM/1(psrSolenoidState) -> psrSolenoidState/1
  FSM/2(psrFsmProfile) -> psrFsmProfile/1

== system Copy_of_eCS_Algo_Simulation_2015b/Input (Pulse// Angle)1/Puls_BMW_KSF_50 ==
  time in : Inport
  Constant : Constant  Value=KSF_50_time
  Constant1 : Constant  Value=KSF_50_a_x
  Constant3 : Constant  Value=KSF_50_a_y
  Lookup Table Dynamic : simulink/Lookup Tables/Lookup Table Dynamic  LookUpMeth=Interpolation-Use End Values  OutDataTypeStr=fixdt('double')  OutputDataTypeScalingMode=Specify via dialog  OutDataType=fixdt('double')  OutScaling=[]  DoSatur=off
  Lookup Table Dynamic1 : simulink/Lookup Tables/Lookup Table Dynamic  LookUpMeth=Interpolation-Use End Values  OutDataTypeStr=fixdt('double')  OutputDataTypeScalingMode=Specify via dialog  OutDataType=fixdt('double')  OutScaling=[]  DoSatur=off
  Mux : Mux  Inputs=2
  Rate Transition1 : RateTransition
  Rate Transition2 : RateTransition  OutPortSampleTime=1/2000
  Scope : Scope
  m/s² to g : Gain  Gain=1/9.81
  pulse out [x,y] (g) : Outport
  wires:
  Lookup Table Dynamic/1 -> Mux/1
  Rate Transition2/1 -> Lookup Table Dynamic1/1, Lookup Table Dynamic/1
  Lookup Table Dynamic1/1 -> Mux/2
  time in/1 -> Rate Transition2/1
  Constant1/1 -> Lookup Table Dynamic/3
  Constant/1 -> Lookup Table Dynamic1/2, Lookup Table Dynamic/2
  Constant3/1 -> Lookup Table Dynamic1/3
  Rate Transition1/1 -> Scope/1, pulse out [x,y] (g)/1
  m/s² to g/1 -> Rate Transition1/1
  Mux/1 -> m/s² to g/1

== system Copy_of_eCS_Algo_Simulation_2015b/Input (Pulse// Angle)1/Puls_BMW_KSG_30 ==
  time in : Inport
  Constant : Constant  Value=KSG_30_time
  Constant1 : Constant  Value=KSG_30_a_x
  Constant3 : Constant  Value=KSG_30_a_y
  Lookup Table Dynamic : simulink/Lookup Tables/Lookup Table Dynamic  LookUpMeth=Interpolation-Use End Values  OutDataTypeStr=fixdt('double')  OutputDataTypeScalingMode=Specify via dialog  OutDataType=fixdt('double')  OutScaling=[]  DoSatur=off
  Lookup Table Dynamic1 : simulink/Lookup Tables/Lookup Table Dynamic  LookUpMeth=Interpolation-Use End Values  OutDataTypeStr=fixdt('double')  OutputDataTypeScalingMode=Specify via dialog  OutDataType=fixdt('double')  OutScaling=[]  DoSatur=off
  Mux : Mux  Inputs=2
  Rate Transition1 : RateTransition
  Rate Transition2 : RateTransition  OutPortSampleTime=1/2000
  Scope : Scope
  m/s² to g : Gain  Gain=1/9.81
  pulse out [x,y] (g) : Outport
  wires:
  Mux/1 -> m/s² to g/1
  m/s² to g/1 -> Rate Transition1/1
  Rate Transition1/1 -> pulse out [x,y] (g)/1, Scope/1
  Constant3/1 -> Lookup Table Dynamic1/3
  Constant/1 -> Lookup Table Dynamic/2, Lookup Table Dynamic1/2
  Constant1/1 -> Lookup Table Dynamic/3
  time in/1 -> Rate Transition2/1
  Lookup Table Dynamic1/1 -> Mux/2
  Rate Transition2/1 -> Lookup Table Dynamic/1, Lookup Table Dynamic1/1
  Lookup Table Dynamic/1 -> Mux/1

== system Copy_of_eCS_Algo_Simulation_2015b/Input (Pulse// Angle)1/Puls_BMW_Rauasphalt_60  ==
  time in : Inport
  Constant : Constant  Value=Rauasphalt_60_time
  Constant1 : Constant  Value=Rauasphalt_60_a_x
  Constant3 : Constant  Value=Rauasphalt_60_a_y
  Lookup Table Dynamic : simulink/Lookup Tables/Lookup Table Dynamic  LookUpMeth=Interpolation-Use End Values  OutDataTypeStr=fixdt('double')  OutputDataTypeScalingMode=Specify via dialog  OutDataType=fixdt('double')  OutScaling=[]  DoSatur=off
  Lookup Table Dynamic1 : simulink/Lookup Tables/Lookup Table Dynamic  LookUpMeth=Interpolation-Use End Values  OutDataTypeStr=fixdt('double')  OutputDataTypeScalingMode=Specify via dialog  OutDataType=fixdt('double')  OutScaling=[]  DoSatur=off
  Mux : Mux  Inputs=2
  Rate Transition1 : RateTransition
  Rate Transition2 : RateTransition  OutPortSampleTime=1/2000
  Scope : Scope
  m/s² to g : Gain  Gain=1/9.81
  pulse out [x,y] (g) : Outport
  wires:
  Lookup Table Dynamic/1 -> Mux/1
  Rate Transition2/1 -> Lookup Table Dynamic1/1, Lookup Table Dynamic/1
  Lookup Table Dynamic1/1 -> Mux/2
  time in/1 -> Rate Transition2/1
  Constant1/1 -> Lookup Table Dynamic/3
  Constant/1 -> Lookup Table Dynamic1/2, Lookup Table Dynamic/2
  Constant3/1 -> Lookup Table Dynamic1/3
  Rate Transition1/1 -> Scope/1, pulse out [x,y] (g)/1
  m/s² to g/1 -> Rate Transition1/1
  Mux/1 -> m/s² to g/1

== system Copy_of_eCS_Algo_Simulation_2015b/Input (Pulse// Angle)1/Puls_GWM_road_C.Morgan ==
  time in : Inport
  Constant : Constant  Value=gmw_roadtime_2kHz
  Constant1 : Constant  Value=gmw_roada_x__m_s__
  Constant3 : Constant  Value=gmw_roada_y__m_s__
  Lookup Table Dynamic : simulink/Lookup Tables/Lookup Table Dynamic  LookUpMeth=Interpolation-Use End Values  OutDataTypeStr=fixdt('double')  OutputDataTypeScalingMode=Specify via dialog  OutDataType=fixdt('double')  OutScaling=[]  DoSatur=off
  Lookup Table Dynamic1 : simulink/Lookup Tables/Lookup Table Dynamic  LookUpMeth=Interpolation-Use End Values  OutDataTypeStr=fixdt('double')  OutputDataTypeScalingMode=Specify via dialog  OutDataType=fixdt('double')  OutScaling=[]  DoSatur=off
  Mux : Mux  Inputs=2
  Rate Transition1 : RateTransition
  Rate Transition2 : RateTransition  OutPortSampleTime=1/2000
  Scope : Scope
  m/s² to g : Gain  Gain=1/9.81
  pulse out [x,y] (g) : Outport
  wires:
  Mux/1 -> m/s² to g/1
  m/s² to g/1 -> Rate Transition1/1
  Rate Transition1/1 -> pulse out [x,y] (g)/1, Scope/1
  Constant3/1 -> Lookup Table Dynamic1/3
  Constant/1 -> Lookup Table Dynamic/2, Lookup Table Dynamic1/2
  Constant1/1 -> Lookup Table Dynamic/3
  time in/1 -> Rate Transition2/1
  Lookup Table Dynamic1/1 -> Mux/2
  Rate Transition2/1 -> Lookup Table Dynamic/1, Lookup Table Dynamic1/1
  Lookup Table Dynamic/1 -> Mux/1

== system Copy_of_eCS_Algo_Simulation_2015b/Input (Pulse// Angle)1/Puls_Kopfsteinpflaster Meldorf Hindenburgstrasse ==
  time in : Inport
  Constant : Constant  Value=Meldorf_HindenburgstraTime__s_
  Constant1 : Constant  Value=Meldorf_HindenburgstraAcceleration_x__m_s_2_
  Constant2 : Constant  Value=Meldorf_HindenburgstraAcceleration_z__m_s_2_
  Constant3 : Constant  Value=Meldorf_HindenburgstraAcceleration_y__m_s_2_
  Gain : Gain  Gain=-1
  Lookup Table Dynamic : simulink/Lookup Tables/Lookup Table Dynamic  LookUpMeth=Interpolation-Use End Values  OutDataTypeStr=fixdt('double')  OutputDataTypeScalingMode=Specify via dialog  OutDataType=fixdt('double')  OutScaling=[]  DoSatur=off
  Lookup Table Dynamic1 : simulink/Lookup Tables/Lookup Table Dynamic  LookUpMeth=Interpolation-Use End Values  OutDataTypeStr=fixdt('double')  OutputDataTypeScalingMode=Specify via dialog  OutDataType=fixdt('double')  OutScaling=[]  DoSatur=off
  Lookup Table Dynamic2 : simulink/Lookup Tables/Lookup Table Dynamic  LookUpMeth=Interpolation-Use End Values  OutDataTypeStr=fixdt('double')  OutputDataTypeScalingMode=Specify via dialog  OutDataType=fixdt('double')  OutScaling=[]  DoSatur=off
  Mux : Mux  Inputs=3
  Rate Transition1 : RateTransition
  Rate Transition2 : RateTransition  OutPortSampleTime=1/500
  Scope : Scope
  m/s² to g : Gain  Gain=1/9.81
  pulse out [x,y] (g) : Outport
  wires:
  Lookup Table Dynamic/1 -> Mux/1
  Rate Transition2/1 -> Lookup Table Dynamic2/1, Lookup Table Dynamic1/1, Lookup Table Dynamic/1
  Lookup Table Dynamic1/1 -> Mux/2
  time in/1 -> Rate Transition2/1
  Constant1/1 -> Lookup Table Dynamic/3
  Constant/1 -> Lookup Table Dynamic2/2, Lookup Table Dynamic1/2, Lookup Table Dynamic/2
  Constant3/1 -> Lookup Table Dynamic1/3
  Rate Transition1/1 -> Scope/1, pulse out [x,y] (g)/1
  m/s² to g/1 -> Rate Transition1/1
  Mux/1 -> m/s² to g/1
  Constant2/1 -> Lookup Table Dynamic2/3
  Lookup Table Dynamic2/1 -> Gain/1
  Gain/1 -> Mux/3

== system Copy_of_eCS_Algo_Simulation_2015b/Input (Pulse// Angle)1/Puls_VW416_Atlas_C.Morgan ==
  time in : Inport
  Constant : Constant  Value=VW_416_2kHztime_2kHz
  Constant1 : Constant  Value=VW_416_2kHza_x_2kHz
  Constant3 : Constant  Value=VW_416_2kHza_y_2kHz
  Lookup Table Dynamic : simulink/Lookup Tables/Lookup Table Dynamic  LookUpMeth=Interpolation-Use End Values  OutDataTypeStr=fixdt('double')  OutputDataTypeScalingMode=Specify via dialog  OutDataType=fixdt('double')  OutScaling=[]  DoSatur=off
  Lookup Table Dynamic1 : simulink/Lookup Tables/Lookup Table Dynamic  LookUpMeth=Interpolation-Use End Values  OutDataTypeStr=fixdt('double')  OutputDataTypeScalingMode=Specify via dialog  OutDataType=fixdt('double')  OutScaling=[]  DoSatur=off
  Mux : Mux  Inputs=2
  Rate Transition1 : RateTransition
  Rate Transition2 : RateTransition  OutPortSampleTime=1/2000
  Scope : Scope
  pulse out [x,y] (g) : Outport
  wires:
  Mux/1 -> Rate Transition1/1
  Rate Transition1/1 -> pulse out [x,y] (g)/1, Scope/1
  Constant3/1 -> Lookup Table Dynamic1/3
  Constant/1 -> Lookup Table Dynamic/2, Lookup Table Dynamic1/2
  Constant1/1 -> Lookup Table Dynamic/3
  time in/1 -> Rate Transition2/1
  Lookup Table Dynamic1/1 -> Mux/2
  Rate Transition2/1 -> Lookup Table Dynamic/1, Lookup Table Dynamic1/1
  Lookup Table Dynamic/1 -> Mux/1

== system Copy_of_eCS_Algo_Simulation_2015b/SAD/Subsystem ==
  prrFsmProfile : Inport
  SAD : Subsystem  Tag=MIL Subsystem  Description=c  mask(MIL Subsystem){}
      settings: CopyFcn=if exist('tl_copyfcn','file'), tl_copyfcn(gcbh); end  NameChangeFcn=if exist('tl_namechangefcn','file'), tl_namechangefcn(gcbh); end  DestroyFcn=if exist('update_tl_main_dlg','file'), update_tl_main_dlg('TL_subs_display'); end
  psrExecutedProfiles : Outport
  wires:
  prrFsmProfile/1 -> SAD/1(prrFsmProfile)
  SAD/1(psrExecutedProfiles) -> psrExecutedProfiles/1

== system Copy_of_eCS_Algo_Simulation_2015b/eCS_Targetlink/Subsystem ==
  Ax (m.s-2) : Inport
  Ay (m.s-2) : Inport  Port=2
  Az (m.s-2) : Inport  Port=3
  eCS_Targetlink : Subsystem  Tag=MIL Subsystem  Description=a  mask(MIL Subsystem){}
      settings: CopyFcn=if exist('tl_copyfcn','file'), tl_copyfcn(gcbh); end  NameChangeFcn=if exist('tl_namechangefcn','file'), tl_namechangefcn(gcbh); end  DestroyFcn=if exist('update_tl_main_dlg','file'), update_tl_main_dlg('TL_subs_display'); end
  sBall : Outport
  b8eCSTrigg : Outport  Port=2
  wires:
  Ax (m.s-2)/1 -> eCS_Targetlink/1(Ax (m.s-2))
  Ay (m.s-2)/1 -> eCS_Targetlink/2(Ay (m.s-2))
  Az (m.s-2)/1 -> eCS_Targetlink/3(Az (m.s-2))
  eCS_Targetlink/1(sBall) -> sBall/1
  eCS_Targetlink/2(b8eCSTrigg) -> b8eCSTrigg/1

== system Copy_of_eCS_Algo_Simulation_2015b/µC Signalverarbeitung und Algorithmus2/Calculate Onset >=Threshold ==
  Acceleration x-Axis[g] : Inport
  Acceleration y-Axis[g] : Inport  Port=2
  Acceleration z-Axis[g] : Inport  Port=3
  Abs : Abs
  Abs1 : Abs
  Abs2 : Abs
  Add : Sum
  Calculate Onset x-Axis : Subsystem
  Calculate Onset y-Axis : Subsystem
  Calculate Onset z-Axis : Subsystem
  Compare to Threshold : simulink/Logic and Bit Operations/Compare To Constant  relop=>=  const=1000  OutDataTypeStr=boolean
  Compare to Threshold1 : simulink/Logic and Bit Operations/Compare To Constant  relop=>=  const=1000  OutDataTypeStr=boolean
  Compare to Threshold2 : simulink/Logic and Bit Operations/Compare To Constant  relop=>=  const=1000  OutDataTypeStr=boolean
  Compare to Threshold3 : simulink/Logic and Bit Operations/Compare To Constant  relop=>=  const=1.9  OutDataTypeStr=boolean
  Logical Operator : Logic  Operator=OR  Inputs=3  AllPortsSameDT=off  OutDataTypeStr=boolean
  Logical Operator1 : Logic  AllPortsSameDT=off  OutDataTypeStr=boolean
  Product : Product
  Product1 : Product
  Scope : Scope  NumInputPorts=3
  Scope1 : Scope  NumInputPorts=3
  Scope2 : Scope
  Scope7 : Scope
  Unit Delay : UnitDelay  SampleTime=1/1000
  no lock / lock [bool] : Outport
  wires:
  Product1/1 -> Add/2
  Compare to Threshold3/1 -> Logical Operator1/1
  Add/1 -> Compare to Threshold3/1
  Acceleration y-Axis[g]/1 -> Product1/2, Product1/1, Calculate Onset y-Axis/1(Acceleration [g])
  Calculate Onset x-Axis/1(Onset [g/s]) -> Scope1/1, Abs/1
  Compare to Threshold1/1 -> Scope/2, Logical Operator/2
  Acceleration x-Axis[g]/1 -> Product/2, Product/1, Calculate Onset x-Axis/1(Acceleration [g])
  Product/1 -> Add/1
  Compare to Threshold/1 -> Scope/1, Logical Operator/1
  Logical Operator1/1 -> no lock / lock [bool]/1
  Abs1/1 -> Compare to Threshold1/1
  Calculate Onset y-Axis/1(Onset [g/s]) -> Scope1/2, Abs1/1
  Abs2/1 -> Compare to Threshold2/1
  Logical Operator/1 -> Scope2/1, Unit Delay/1
  Compare to Threshold2/1 -> Scope/3, Logical Operator/3
  Acceleration z-Axis[g]/1 -> Calculate Onset z-Axis/1(Acceleration [g])
  Unit Delay/1 -> Scope7/1, Logical Operator1/2
  Abs/1 -> Compare to Threshold/1
  Calculate Onset z-Axis/1(Onset [g/s]) -> Scope1/3, Abs2/1

== system Copy_of_eCS_Algo_Simulation_2015b/µC Signalverarbeitung und Algorithmus2/Resulting xy >= Threshold ==
  Acceleration x-Axis corrected [g] : Inport
  Acceleration y-Axis corrected [g] : Inport  Port=2
  Add : Sum
  Compare to Threshold : simulink/Logic and Bit Operations/Compare To Constant  relop=>=  const=0.360000000000000  OutDataTypeStr=boolean
  Product : Product
  Product1 : Product
  Sqrt : Sqrt  SaturateOnIntegerOverflow=on
  no lock / lock [bool] : Outport
  wires:
  Compare to Threshold/1 -> no lock / lock [bool]/1
  Sqrt/1 -> Compare to Threshold/1
  Product/1 -> Add/1
  Product1/1 -> Add/2
  Add/1 -> Sqrt/1
  Acceleration x-Axis corrected [g]/1 -> Product/2, Product/1
  Acceleration y-Axis corrected [g]/1 -> Product1/1, Product1/2

== system Copy_of_eCS_Algo_Simulation_2015b/µC Signalverarbeitung und Algorithmus2/Tilt Sensitivity >= Threshold ==
  Acceleration x [g] : Inport
  Acceleration y [g] : Inport  Port=2
  Add : Sum
  Compare to Threshold : simulink/Logic and Bit Operations/Compare To Constant  relop=>=  const=0.358367949545300  OutDataTypeStr=boolean
  Product : Product
  Product1 : Product
  Sqrt : Sqrt  SaturateOnIntegerOverflow=on
  no lock / lock [bool] : Outport
  wires:
  Sqrt/1 -> Compare to Threshold/1
  Product/1 -> Add/1
  Add/1 -> Sqrt/1
  Compare to Threshold/1 -> no lock / lock [bool]/1
  Acceleration x [g]/1 -> Product/2, Product/1
  Acceleration y [g]/1 -> Product1/2, Product1/1
  Product1/1 -> Add/2

== system Copy_of_eCS_Algo_Simulation_2015b/FSM/Subsystem/FSM ==
  prrEcsAlgoFlag : Inport
      settings: NameChangeFcn=if exist('tl_check_ports','file'), tl_check_ports(gcbh); end
      settings: CopyFcn=|
      | if exist('tl_reset_reviewflag','file')==2
      |     tl_reset_reviewflag(gcbh);
      | end
      | if exist('tl_check_ports','file')
      |     tl_check_ports(gcbh);
      | end
  prrVehicleInputs : Inport  Port=2
      settings: NameChangeFcn=if exist('tl_check_ports','file'), tl_check_ports(gcbh); end
      settings: CopyFcn=|
      | if exist('tl_reset_reviewflag','file')==2
      |     tl_reset_reviewflag(gcbh);
      | end
      | if exist('tl_check_ports','file')
      |     tl_check_ports(gcbh);
      | end
  prrExecutedProfiles : Inport  Port=3
      settings: NameChangeFcn=if exist('tl_check_ports','file'), tl_check_ports(gcbh); end
      settings: CopyFcn=|
      | if exist('tl_reset_reviewflag','file')==2
      |     tl_reset_reviewflag(gcbh);
      | end
      | if exist('tl_check_ports','file')
      |     tl_check_ports(gcbh);
      | end
  FSM : Subsystem
  psrSolenoidState : Outport
      settings: NameChangeFcn=if exist('tl_check_ports','file'), tl_check_ports(gcbh); end
      settings: CopyFcn=|
      | if exist('tl_reset_reviewflag','file')==2
      |     tl_reset_reviewflag(gcbh);
      | end
      | if exist('tl_check_ports','file')
      |     tl_check_ports(gcbh);
      | end
  psrFsmProfile : Outport  Port=2
      settings: NameChangeFcn=if exist('tl_check_ports','file'), tl_check_ports(gcbh); end
      settings: CopyFcn=|
      | if exist('tl_reset_reviewflag','file')==2
      |     tl_reset_reviewflag(gcbh);
      | end
      | if exist('tl_check_ports','file')
      |     tl_check_ports(gcbh);
      | end
  wires:
  prrEcsAlgoFlag/1 -> FSM/1(prrEcsAlgoFlag)
  prrVehicleInputs/1 -> FSM/2(prrVehicleInputs)
  FSM/1(psrSolenoidState) -> psrSolenoidState/1
  FSM/2(psrFsmProfile) -> psrFsmProfile/1
  prrExecutedProfiles/1 -> FSM/3(prrExecutedProfiles)

== system Copy_of_eCS_Algo_Simulation_2015b/SAD/Subsystem/SAD ==
  prrFsmProfile : Inport
      settings: NameChangeFcn=if exist('tl_check_ports','file'), tl_check_ports(gcbh); end
      settings: CopyFcn=|
      | if exist('tl_reset_reviewflag','file')==2
      |     tl_reset_reviewflag(gcbh);
      | end
      | if exist('tl_check_ports','file')
      |     tl_check_ports(gcbh);
      | end
  SAD : Subsystem
  psrExecutedProfiles : Outport  mask(TL_BusOutport){data={'#autoscaling',2,'#message',2,'#output',2,'#logdata',2,'logdata#1',{'loggingmode',1},'output#1',{'type','AUTOLIV/FSM_DataDictionnary/ImplementationDataTypes/au8FsmProfileType','scaling','AUTOLIV/FSM_DataDictionnary/ComputationMethods/scFsmProfiles'},'output#2',{'type','AUTOLIV/FSM_DataDictionnary/ImplementationDataTypes/au8FsmProfileType','scaling','AUTOLIV/FSM_DataDictionnary/ComputationMethods/scFsmProfiles'},'signals',{{'isrExecutedProfile',{'u8ExecutedProfile';'u8ExecutedProfileOld'}}},'date',738344.6860284491}}
      settings: DeleteFcn=if exist('delete_tlblock','file')==2,delete_tlblock(gcbh);end  OpenFcn=if exist('tl_open_blockdlg','file')==2,tl_open_blockdlg(gcbh);else,open_system(gcbh,'parameter');end
      settings: CopyFcn=|
      | if exist('tl_reset_reviewflag','file')==2
      |     tl_reset_reviewflag(gcbh);
      | end
      | if exist('tl_check_ports','file')
      |     tl_check_ports(gcbh);
      | end
      settings: NameChangeFcn=|
      | if exist('rename_tlblock','file')==2,rename_tlblock(gcbh);end
      | if exist('tl_check_ports','file'), tl_check_ports(gcbh); end
      mask Help: eval(['if exist(''tl_online_help'',''file'') == 2, tl_online_help(''Topic'',''TL_Outport''),else, web([''jar:file:///'',matlabroot,''/help/toolbox/simulink/help.jar!/slref/' lower(get_param(gcbh,'Blocktype')) '.html''], ''-helpbrowser''),end'])
      mask Display: plot([0.2 0.35 NaN 0.65 0.8],[0 1 NaN 0 1]);
  wires:
  SAD/1(psrExecutedProfiles) -> psrExecutedProfiles/1
  prrFsmProfile/1 -> SAD/1(prrFsmProfile)
